simulink model "PID_DOB_sim"  (R2023b)
settings: Solver=VariableStepAuto  StartTime=0.0  StopTime=2  RelTol=1e-3
values from neighbouring files (symbols this model uses):
  Beq = Jeq/t    (= 0.00264630474582)    [PID_DOB.m]
  Beq_L = Beq+((Kg^2)*B_l/a)    (= 0.00468909971272)    [PID_DOB.m]
  Jeq = J + Kg^2/a*Jg    (= 9.9501058443e-06)    [PID_DOB.m]
  Jeq_L = Jeq+((Kg^2)*J_l/a)    (= 1.76310149198e-05)    [PID_DOB.m]
  Ka_c = 1/Kp_c    (= 1.20941973492)    [PID_DOB.m]
  Ka_s = 1/Kp_s    (= 0.380593455832)    [PID_DOB.m]
  Kd_p = wcp/wcs    (= 0.1)    [PID_DOB.m]
  Ke = Kt    (= 0.0683)    [PID_DOB.m]
  Kg = 1/81    (= 0.0123456790123)    [PID_DOB.m]
  Ki_c = Ra*wcc    (= 2211.616)    [PID_DOB.m]
  Ki_s = Beq_L*wcs/Kt*81    (= 698.796689047)    [PID_DOB.m]
  Kp_c = La*wcc    (= 0.8268428)    [PID_DOB.m]
  Kp_p = wcp    (= 12.566)    [PID_DOB.m]
  Kp_s = Jeq_L*wcs/Kt*81    (= 2.62747555082)    [PID_DOB.m]
  Kt = 68.3*10^-3    (= 0.0683)    [PID_DOB.m]
  La = 0.658*10^-3    (= 0.000658)    [PID_DOB.m]
  Ra = 1.76    [PID_DOB.m]
  tau = 0.001    [PID_DOB.m]
undefined symbols (not defined in the file or in its folder): X, Y, Z
libraries: sm_lib x8, nesl_utility x4
settings Model: Creator=OWNER  LastModifiedBy=Magnetic_Robotics
settings DebuggingCC: UnconnectedInputMsg=warning  UnconnectedOutputMsg=warning  UnconnectedLineMsg=warning
settings ModelReferenceCC: EnableRefExpFcnMdlSchedulingChecks=on
settings RTWCC: DLArmComputeVersion=19.05

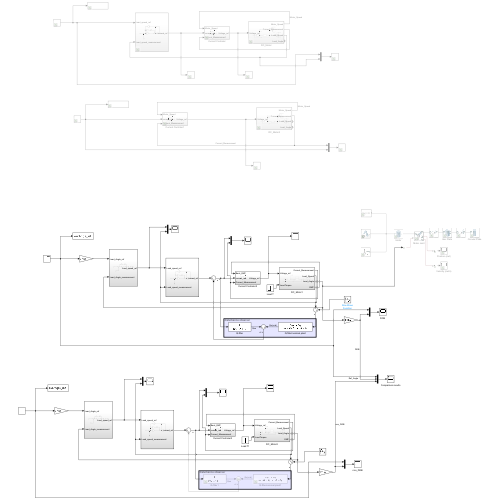
[thumbnail: Simulink's stored preview of the top-level diagram]
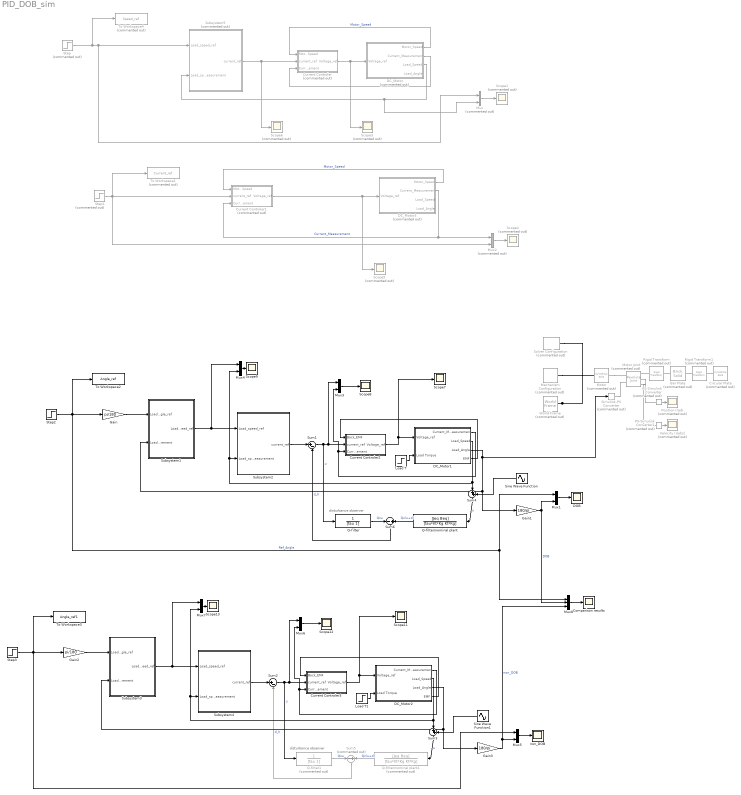
== system PID_DOB_sim ==
  note: disturbance observer
  note: disturbance observer
  Bar Plate : sm_lib/Body Elements/Brick Solid  Commented=on  GraphicAmbientColor=[0.15 0.15 0.15 1.0]  BasedOnType=Mass  BrickDimensions=[10 25 300]  BrickDimensionsUnits=mm  CenterOfMass=[0 0 0]  CenterOfMassUnits=m  GraphicDiffuseColor=[1.0 0.2 0.2]  Density=1000  DensityUnits=kg/m^3  DoExposeReferenceFrame=off  GraphicEmissiveColor=[0.0 0.0 0.0 1.0]  ExportEntireGeometry=off  SerializedFrames=<Frames><Frame><Id>Frame1</Id><Value><Name>F1</Name><Origin><Source>GeometricFeature</Source><FeatureName>-z surface</FeatureName></Origin><PrimaryAxis><DefinedDirection>+X</DefinedDirection><Source>ReferenceFrame</Source><SourceDirection>+Z</SourceDirection><FeatureName></FeatureName></PrimaryAxis><SecondaryAxis><DefinedDirection>+Z</DefinedDirection><Source>ReferenceFrame</Source><SourceDirection>+X</SourceDirection><FeatureName></FeatureName></SecondaryAxis></Value></Frame><Frame><Id>Frame2</Id><Value><Name>F2</Name><Origin><Source>GeometricFeature</Source><FeatureName>+z surface</FeatureName></Origin><PrimaryAxis><DefinedDirection>+Y</DefinedDirection><Source>ReferenceFrame</Source><SourceDirection>+Z</SourceDirection><FeatureName></FeatureName></PrimaryAxis><SecondaryAxis><DefinedDirection>+Z</DefinedDirection><Source>ReferenceFrame</Source><SourceDirection>+X</SourceDirection><FeatureName></FeatureName></SecondaryAxis></Value></Frame></Frames>  MarkerShape=Sphere  MarkerSize=10  GraphicType=FromGeometry  InertiaType=CalculateFromGeometry  Mass=175  MassUnits=g  MomentsOfInertia=[1 1 1]  MomentsOfInertiaUnits=kg*m^2  GraphicOpacity=1.0  ProductsOfInertia=[0 0 0]  ProductsOfInertiaUnits=kg*m^2  GraphicShininess=75  GraphicSpecularColor=[0.5 0.5 0.5 1.0]  GraphicVisPropType=SimpleVisualProperties
  Circular Plate : sm_lib/Body Elements/Cylindrical Solid  Commented=on  GraphicAmbientColor=[0.15 0.15 0.15 1.0]  BasedOnType=Mass  CenterOfMass=[0 0 0]  CenterOfMassUnits=m  GraphicDiffuseColor=[1.0 0.0 0.8]  CylinderLength=10  CylinderLengthUnits=mm  CylinderRadius=50  CylinderRadiusUnits=mm  Density=1000  DensityUnits=kg/m^3  DoExposeReferenceFrame=off  GraphicEmissiveColor=[0.0 0.0 0.0 1.0]  ExportEntireGeometry=off  SerializedFrames=<Frames><Frame><Id>Frame1</Id><Value><Name>F1</Name><Origin><Source>ReferenceFrame</Source><FeatureName></FeatureName></Origin><PrimaryAxis><DefinedDirection>+Z</DefinedDirection><Source>ReferenceFrame</Source><SourceDirection>+Z</SourceDirection><FeatureName></FeatureName></PrimaryAxis><SecondaryAxis><DefinedDirection>+X</DefinedDirection><Source>ReferenceFrame</Source><SourceDirection>+X</SourceDirection><FeatureName></FeatureName></SecondaryAxis></Value></Frame></Frames>  MarkerShape=Sphere  MarkerSize=10  GraphicType=FromGeometry  InertiaType=CalculateFromGeometry  Mass=340  MassUnits=g  MomentsOfInertia=[1 1 1]  MomentsOfInertiaUnits=kg*m^2  GraphicOpacity=1.0  ProductsOfInertia=[0 0 0]  ProductsOfInertiaUnits=kg*m^2  GraphicShininess=75  GraphicSpecularColor=[0.5 0.5 0.5 1.0]  GraphicVisPropType=SimpleVisualProperties
  Comparison results : Scope
  Current Controler : Subsystem  Commented=on
  Current Controler1 : Subsystem  Commented=on
  Current Controler2 : Subsystem
  Current Controler3 : Subsystem
  DC_Motor : Subsystem  Commented=on
  DC_Motor1 : Subsystem
  DC_Motor2 : Subsystem
  DC_Motor3 : Subsystem  Commented=on
  DOB : Scope
  Gain : Gain  Gain=pi/180
  Gain1 : Gain  Gain=180/pi
  Gain2 : Gain  Gain=pi/180
  Gain3 : Gain  Gain=180/pi
  Load T : Step  Time=0.1  After=2  SampleTime=0
  Load T1 : Step  Time=0.1  After=2  SampleTime=0
  Mechanism Configuration : sm_lib/Utilities/Mechanism Configuration  Commented=on  UniformGravity=Constant  GravityVector=[0 0 -9.80665]  GravityVectorUnits=m/s^2  LinearizationDelta=0.001  JointModeTransitionNonlinearIterations=2
  Motor : sm_lib/Body Elements/Cylindrical Solid  Commented=on  GraphicAmbientColor=[0.15 0.15 0.15 1.0]  BasedOnType=Density  CenterOfMass=[0 0 0]  CenterOfMassUnits=m  GraphicDiffuseColor=[0.5 0.5 0.5]  CylinderLength=150  CylinderLengthUnits=mm  CylinderRadius=30  CylinderRadiusUnits=mm  Density=1000  DensityUnits=kg/m^3  DoExposeReferenceFrame=off  GraphicEmissiveColor=[0.0 0.0 0.0 1.0]  ExportEntireGeometry=off  SerializedFrames=<Frames><Frame><Id>Frame1</Id><Value><Name>F1</Name><Origin><Source>ReferenceFrame</Source><FeatureName></FeatureName></Origin><PrimaryAxis><DefinedDirection>+Z</DefinedDirection><Source>ReferenceFrame</Source><SourceDirection>+Z</SourceDirection><FeatureName></FeatureName></PrimaryAxis><SecondaryAxis><DefinedDirection>+X</DefinedDirection><Source>ReferenceFrame</Source><SourceDirection>+X</SourceDirection><FeatureName></FeatureName></SecondaryAxis></Value></Frame><Frame><Id>Frame2</Id><Value><Name>F2</Name><Origin><Source>GeometricFeature</Source><FeatureName>top surface</FeatureName></Origin><PrimaryAxis><DefinedDirection>+Z</DefinedDirection><Source>ReferenceFrame</Source><SourceDirection>+Z</SourceDirection><FeatureName></FeatureName></PrimaryAxis><SecondaryAxis><DefinedDirection>+X</DefinedDirection><Source>ReferenceFrame</Source><SourceDirection>+X</SourceDirection><FeatureName></FeatureName></SecondaryAxis></Value></Frame></Frames>  MarkerShape=Sphere  MarkerSize=10  GraphicType=FromGeometry  InertiaType=CalculateFromGeometry  Mass=1  MassUnits=kg  MomentsOfInertia=[1 1 1]  MomentsOfInertiaUnits=kg*m^2  GraphicOpacity=1.0  ProductsOfInertia=[0 0 0]  ProductsOfInertiaUnits=kg*m^2  GraphicShininess=75  GraphicSpecularColor=[0.5 0.5 0.5 1.0]  GraphicVisPropType=SimpleVisualProperties
  Motor Joint : sm_lib/Joints/Revolute Joint  Commented=on  JointMode=Normal  SenseConstraintForce=off  SenseConstraintForceX=off  SenseConstraintForceY=off  SenseConstraintForceZ=off  SenseConstraintTorque=off  SenseConstraintTorqueX=off  SenseConstraintTorqueY=off  SenseConstraintTorqueZ=off  SenseTotalForce=off  SenseTotalForceX=off  SenseTotalForceY=off  SenseTotalForceZ=off  SenseTotalTorque=off  SenseTotalTorqueX=off  SenseTotalTorqueY=off  SenseTotalTorqueZ=off  CompositeWrenchDir=FollowerOnBase  CompositeWrenchFrame=BaseFrame  EquilibriumPosition=0  EquilibriumPositionUnits=deg  SpringStiffness=0  SpringStiffnessUnits=N*m/deg  DampingCoefficient=0  DampingCoefficientUnits=N*m/(deg/s)  TorqueActuationMode=ComputedTorque  MotionActuationMode=InputMotion  SensePosition=on  SenseVelocity=on  SenseAcceleration=off  SenseTorqueForce=off  SenseLowerLimitTorqueForce=off  SenseUpperLimitTorqueForce=off  LowerLimitSpecify=off  LowerLimitBound=-90  LowerLimitBoundUnits=deg  LowerLimitStiffness=1e4  LowerLimitStiffnessUnits=N*m/deg  LowerLimitDamping=10  LowerLimitDampingUnits=N*m/(deg/s)  LowerLimitTransitionRegionWidth=0.1  LowerLimitTransitionRegionWidthUnits=deg  UpperLimitSpecify=off  UpperLimitBound=90  UpperLimitBoundUnits=deg  UpperLimitStiffness=1e4  UpperLimitStiffnessUnits=N*m/deg  UpperLimitDamping=10  UpperLimitDampingUnits=N*m/(deg/s)  UpperLimitTransitionRegionWidth=0.1  UpperLimitTransitionRegionWidthUnits=deg  PositionTargetSpecify=off  PositionTargetPriority=High  PositionTargetValue=0  PositionTargetValueUnits=deg  VelocityTargetSpecify=off  VelocityTargetPriority=High  VelocityTargetValue=0  VelocityTargetValueUnits=deg/s
  Mux : Mux  Commented=on  Inputs=2
  Mux{1,3..7} (6 alike) : Mux  Inputs=2
  Mux2 : Mux  Commented=on  Inputs=2
  Mux8 : Mux  Inputs=3
  PS-Simulink Converter : nesl_utility/PS-Simulink Converter  Commented=on  PhysicalDomain=network_engine_domain  SubClassName=ps_output  LeftPortType=input  RightPortType=output  PseudoPeriodic=off  Frequencies=[]  VectorFormat=1-D array  Unit=inherit  AffineConversion=off
  PS-Simulink Converter1 : nesl_utility/PS-Simulink Converter  Commented=on  PhysicalDomain=network_engine_domain  SubClassName=ps_output  LeftPortType=input  RightPortType=output  PseudoPeriodic=off  Frequencies=[]  VectorFormat=1-D array  Unit=inherit  AffineConversion=off
  Position (rad) : Scope  Commented=on
  Q-filter : TransferFcn  Denominator=[tau 1]
  Q-filter/nominal plant : TransferFcn  Numerator=[Jeq Beq]  Denominator=[tau*Kt*Kg Kt*Kg]
  Q-filter/nominal plant1 : TransferFcn  Commented=on  Numerator=[Jeq Beq]  Denominator=[tau*Kt*Kg Kt*Kg]
  Q-filter1 : TransferFcn  Commented=on  Denominator=[tau 1]
  Rigid Transform : sm_lib/Frames and Transforms/Rigid Transform  Commented=on  TranslationMethod=StandardAxis  TranslationStandardOffset=5  TranslationStandardOffsetUnits=mm  TranslationStandardAxis=+Z  TranslationCartesianOffset=[0 0 0]  TranslationCartesianOffsetUnits=mm  TranslationROffset=0  TranslationROffsetUnits=m  TranslationZOffset=0  TranslationZOffsetUnits=m  TranslationThetaOffset=0  TranslationThetaOffsetUnits=deg  RotationMethod=None  RotationAngleUnits=deg  RotationStandardAxis=+Z  RotationAngle=0.0  RotationArbitraryAxis=[0 0 1]  FollAlignAxisA=+X  BaseAlignAxisA=+Y  FollAlignAxisB=+Y  BaseAlignAxisB=+Z  RotationSequenceAxes=FollowerAxes  RotationSequence=XYX  RotationSequenceAngles=[0 0 0]  RotationSequenceAnglesUnits=deg  RotationMatrix=[1 0 0; 0 1 0; 0 0 1]  Quaternion=[1 0 0 0]
  Rigid Transform1 : sm_lib/Frames and Transforms/Rigid Transform  Commented=on  TranslationMethod=StandardAxis  TranslationStandardOffset=10  TranslationStandardOffsetUnits=mm  TranslationStandardAxis=+Z  TranslationCartesianOffset=[0 0 0]  TranslationCartesianOffsetUnits=mm  TranslationROffset=0  TranslationROffsetUnits=m  TranslationZOffset=0  TranslationZOffsetUnits=m  TranslationThetaOffset=0  TranslationThetaOffsetUnits=deg  RotationMethod=None  RotationAngleUnits=deg  RotationStandardAxis=+Z  RotationAngle=0.0  RotationArbitraryAxis=[0 0 1]  FollAlignAxisA=+X  BaseAlignAxisA=+Y  FollAlignAxisB=+Y  BaseAlignAxisB=+Z  RotationSequenceAxes=FollowerAxes  RotationSequence=XYX  RotationSequenceAngles=[0 0 0]  RotationSequenceAnglesUnits=deg  RotationMatrix=[1 0 0; 0 1 0; 0 0 1]  Quaternion=[1 0 0 0]
  Scope{1,3..6} (5 alike) : Scope  Commented=on
  Scope{7..9,11..13} (6 alike) : Scope
  Simulink-PS Converter : nesl_utility/Simulink-PS Converter  Commented=on  PhysicalDomain=network_engine_domain  SubClassName=ps_input  LeftPortType=input  RightPortType=output  PseudoPeriodic=off  Frequencies=[]  NoiseDistribution=none  NoiseParameters=[]  Unit=rad  AffineConversion=off  FilteringAndDerivatives=filter  SimscapeFilterOrder=2  InputFilterTimeConstant=0.001  UdotUserProvided=0
  Sine Wave Function : Sin  Frequency=10  SampleTime=0
  Sine Wave Function1 : Sin  Frequency=10  SampleTime=0
  Solver Configuration : nesl_utility/Solver Configuration  Commented=on  PhysicalDomain=network_engine_domain  SubClassName=solver  LeftPortType=input  RightPortType=generic  Tones=[]  Harmonics=[]  SimulateNoise=off  Profile=off  UseLocalSampling=off  EnableSwitchedLinearOptims=on  FrequencyDomain=off  UseCCode=off  RelTol=0.001  AbsTol=0.001  MinStep=1e-09  ToWorkspace=off  RevertToSquareIcSolve=off  NumHomotopyIterations=100  PhasorMode=off  PhasorModeNumHarmonics=1  ConsistencySolver=NEWTON_FTOL  IndexReductionMethod=DerivativeReplacement  DoDC=off  ResidualTolerance=1e-09  ConsistencyTolSource=GLOBAL  ConsistencyAbsTol=0.001  ConsistencyRelTol=0.001  ConsistencyTolFactor=0.001  UseLocalSolver=off  LocalSolverChoice=NE_BACKWARD_EULER_ADVANCER  ResolveIndetEquations=on  FunctionEvalNumThread=1  LocalSolverSampleTime=0.001  DoFixedCost=off  MaxNonlinIter=3  MaxModeIter=2  ComputeImpulses=off  ImpulseIterations=2  LinearAlgebra=auto  LinearAlgebraNumThread=0  EquationFormulation=NE_TIME_EF  DelaysMemoryBudget=1024  AutomaticFiltering=on  FilteringTimeConstant=0.001  PartitionStorageMethod=AS_NEEDED  PartitionMemoryBudget=1024  PartitionMethod=ROBUST  MultibodyUseLocalSolver=off  MultibodyLocalSolverChoice=ODE1  MultibodyLocalSolverSampleTime=0.001
  Step : Step  Commented=on  Before=5  After=5  SampleTime=0
  Step1 : Step  Commented=on  Before=25  After=25  SampleTime=0
  Step2 : Step  Time=0.1  After=60  SampleTime=0
  Step3 : Step  Time=0.1  After=60  SampleTime=0
  Subsystem1 : Subsystem
  Subsystem2 : Subsystem
  Subsystem3 : Subsystem
  Subsystem4 : Subsystem
  Subsystem5 : Subsystem  Commented=on
  Sum1 : Sum  Inputs=|+-
  Sum2 : Sum  Inputs=|+-
  Sum3 : Sum  Inputs=|++
  Sum4 : Sum  Inputs=|++
  Sum5 : Sum  Commented=on  Inputs=-|+
  Sum6 : Sum  Inputs=-|+
  To Workspace1 : ToWorkspace  Commented=on  VariableName=Current_ref  SaveFormat=Structure With Time  SampleTime=-1
  To Workspace2 : ToWorkspace  VariableName=Angle_ref  SaveFormat=Structure With Time  SampleTime=-1
  To Workspace3 : ToWorkspace  VariableName=Angle_ref1  SaveFormat=Structure With Time  SampleTime=-1
  To Workspace4 : ToWorkspace  Commented=on  VariableName=Speed_ref  SaveFormat=Structure With Time  SampleTime=-1
  Velocity (rad/s) : Scope  Commented=on
  World Frame : sm_lib/Frames and Transforms/World Frame  Commented=on
  non_DOB : Scope
  wires:
  DC_Motor/1(Motor_Speed) -> Current Controler/1(Motor_Speed)  "Motor_Speed"
  Step/1 -> To Workspace4/1, Mux/1, Subsystem5/1(Load_speed_ref)
  Current Controler/1(Voltage_ref) -> Scope3/1, DC_Motor/1(Voltage_ref)
  Mux/1 -> Scope1/1
  Step1/1 -> To Workspace1/1, Mux2/2, Current Controler1/2(current_ref)
  Mux2/1 -> Scope4/1
  Current Controler1/1(Voltage_ref) -> Scope5/1, DC_Motor3/1(Voltage_ref)
  DC_Motor3/2(Current_Measurement) -> Mux2/1, Current Controler1/3(Current_Measurement)  "Current_Measurement"
  DC_Motor3/1(Motor_Speed) -> Current Controler1/1(Motor_Speed)  "Motor_Speed"
  DC_Motor/2(Current_Measurement) -> Current Controler/3(Current_Measurement)
  DC_Motor/3(Load_Speed) -> Mux/2, Subsystem5/2(Load_speed_measurement)
  Subsystem5/1(current_ref) -> Scope6/1, Current Controler/2(current_ref)
  Subsystem2/1(current_ref) -> Sum1/1
  DC_Motor1/2(Load_Speed) -> Sum4/1, Mux4/2, Subsystem2/2(Load_speed_measurement)
  Step2/1 -> Gain/1, Mux8/1, Mux1/1, To Workspace2/1  "Ref_Angle"
  Mux1/1 -> DOB/1
  Gain/1 -> Subsystem1/1(Load_Angle_ref)
  Gain1/1 -> Mux8/2, Mux1/2  "DOB"
  Subsystem1/1(Load_speed_ref) -> Subsystem2/1(Load_speed_ref), Mux4/1
  PS-Simulink Converter1/1 -> Velocity (rad/s)/1
  PS-Simulink Converter/1 -> Position (rad)/1
  Sum6/1 -> Sum1/2  "d_h"
  Q-filter/1 -> Sum6/1  "Qxu"
  Q-filter/nominal plant/1 -> Sum6/2  "Qx(u+d)"
  Sum1/1 -> Q-filter/1, Mux3/1, Current Controler2/2(current_ref)  "u"
  DC_Motor1/3(Load_Angle) -> Gain1/1, Subsystem1/2(Load_Angle_measurement), Simulink-PS Converter/1
  Load T/1 -> DC_Motor1/2(Load Torque)
  DC_Motor1/4(EMF) -> Current Controler2/1(Back_EMF)
  Current Controler2/1(Voltage_ref) -> Scope7/1, DC_Motor1/1(Voltage_ref)
  DC_Motor1/1(Current_Measurement) -> Mux3/2, Current Controler2/3(Current_Measurement)
  Mux3/1 -> Scope8/1
  Mux4/1 -> Scope9/1
  Sum4/1 -> Q-filter/nominal plant/1  "u"
  Sine Wave Function/1 -> Sum4/2
  Sine Wave Function1/1 -> Sum3/2
  Sum5/1 -> Sum2/2  "d_h"
  Q-filter/nominal plant1/1 -> Sum5/2  "Qx(u+d)"
  Sum3/1 -> Q-filter/nominal plant1/1  "u"
  Current Controler3/1(Voltage_ref) -> Scope11/1, DC_Motor2/1(Voltage_ref)
  Mux6/1 -> Scope12/1
  DC_Motor2/1(Current_Measurement) -> Mux6/2, Current Controler3/3(Current_Measurement)
  Load T1/1 -> DC_Motor2/2(Load Torque)
  Subsystem4/1(current_ref) -> Sum2/1
  DC_Motor2/2(Load_Speed) -> Sum3/1, Mux7/2, Subsystem4/2(Load_speed_measurement)
  DC_Motor2/3(Load_Angle) -> Gain3/1, Subsystem3/2(Load_Angle_measurement)
  Sum2/1 -> Q-filter1/1, Mux6/1, Current Controler3/2(current_ref)  "u"
  Q-filter1/1 -> Sum5/1  "Qxu"
  DC_Motor2/4(EMF) -> Current Controler3/1(Back_EMF)
  Step3/1 -> Gain2/1, Mux5/1, To Workspace3/1
  Subsystem3/1(Load_speed_ref) -> Subsystem4/1(Load_speed_ref), Mux7/1
  Mux5/1 -> non_DOB/1
  Mux7/1 -> Scope13/1
  Gain2/1 -> Subsystem3/1(Load_Angle_ref)
  Gain3/1 -> Mux8/3, Mux5/2  "non_DOB"
  Mux8/1 -> Comparison results/1
  connections:
  World Frame/RConn1 -- Solver Configuration/RConn1 -- Motor/LConn1 -- Mechanism Configuration/RConn1
  Circular Plate/LConn1 -- Rigid Transform1/RConn1
  Motor/RConn1 -- Motor Joint/LConn1
  Motor Joint/RConn2 -- PS-Simulink Converter/LConn1
  Bar Plate/LConn1 -- Rigid Transform/RConn1
  Rigid Transform1/LConn1 -- Bar Plate/RConn1
  Simulink-PS Converter/RConn1 -- Motor Joint/LConn2
  Rigid Transform/LConn1 -- Motor Joint/RConn1
  Motor Joint/RConn3 -- PS-Simulink Converter1/LConn1

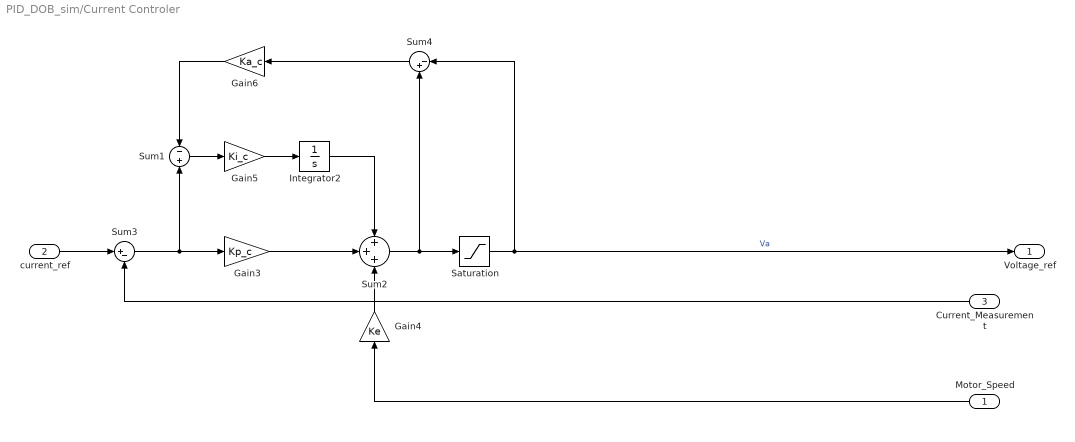
== system PID_DOB_sim/Current Controler ==
  Motor_Speed : Inport
  current_ref : Inport  Port=2
  Current_Measurement : Inport  Port=3
  Gain3 : Gain  Gain=Kp_c
  Gain4 : Gain  Gain=Ke
  Gain5 : Gain  Gain=Ki_c
  Gain6 : Gain  Gain=Ka_c
  Integrator2 : Integrator
  Saturation : Saturate  UpperLimit=48  LowerLimit=-48
  Sum1 : Sum  Inputs=-+
  Sum2 : Sum  Inputs=+++
  Sum3 : Sum  Inputs=|+-
  Sum4 : Sum  Inputs=|-+
  Voltage_ref : Outport
  wires:
  Gain6/1 -> Sum1/1
  Saturation/1 -> Voltage_ref/1, Sum4/1  "Va"
  Sum4/1 -> Gain6/1
  Sum1/1 -> Gain5/1
  Current_Measurement/1 -> Sum3/2
  Integrator2/1 -> Sum2/1
  Sum2/1 -> Sum4/2, Saturation/1
  Gain3/1 -> Sum2/2
  Gain4/1 -> Sum2/3
  Sum3/1 -> Sum1/2, Gain3/1
  Motor_Speed/1 -> Gain4/1
  Gain5/1 -> Integrator2/1
  current_ref/1 -> Sum3/1

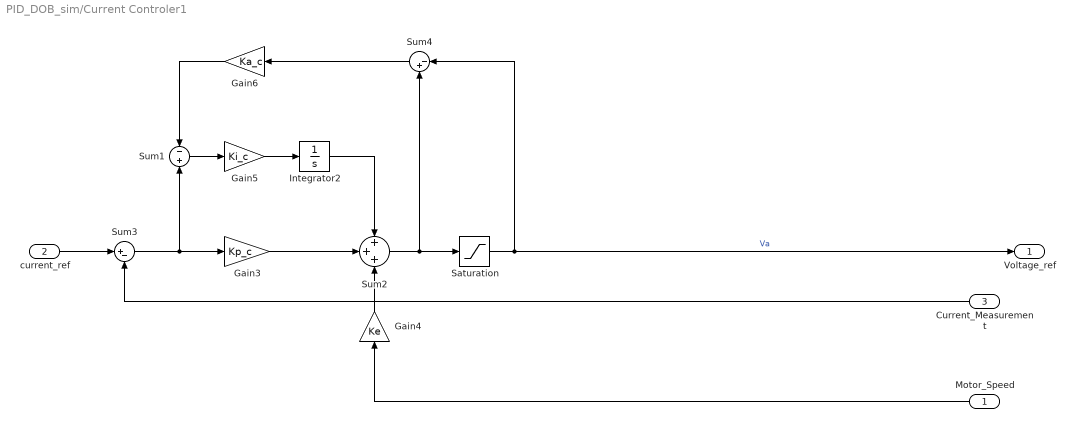
== system PID_DOB_sim/Current Controler1 ==
  Motor_Speed : Inport
  current_ref : Inport  Port=2
  Current_Measurement : Inport  Port=3
  Gain3 : Gain  Gain=Kp_c
  Gain4 : Gain  Gain=Ke
  Gain5 : Gain  Gain=Ki_c
  Gain6 : Gain  Gain=Ka_c
  Integrator2 : Integrator
  Saturation : Saturate  UpperLimit=48  LowerLimit=-48
  Sum1 : Sum  Inputs=-+
  Sum2 : Sum  Inputs=+++
  Sum3 : Sum  Inputs=|+-
  Sum4 : Sum  Inputs=|-+
  Voltage_ref : Outport
  wires:
  Gain6/1 -> Sum1/1
  Saturation/1 -> Voltage_ref/1, Sum4/1  "Va"
  Sum4/1 -> Gain6/1
  Sum1/1 -> Gain5/1
  Current_Measurement/1 -> Sum3/2
  Integrator2/1 -> Sum2/1
  Sum2/1 -> Sum4/2, Saturation/1
  Gain3/1 -> Sum2/2
  Gain4/1 -> Sum2/3
  Sum3/1 -> Sum1/2, Gain3/1
  Motor_Speed/1 -> Gain4/1
  Gain5/1 -> Integrator2/1
  current_ref/1 -> Sum3/1

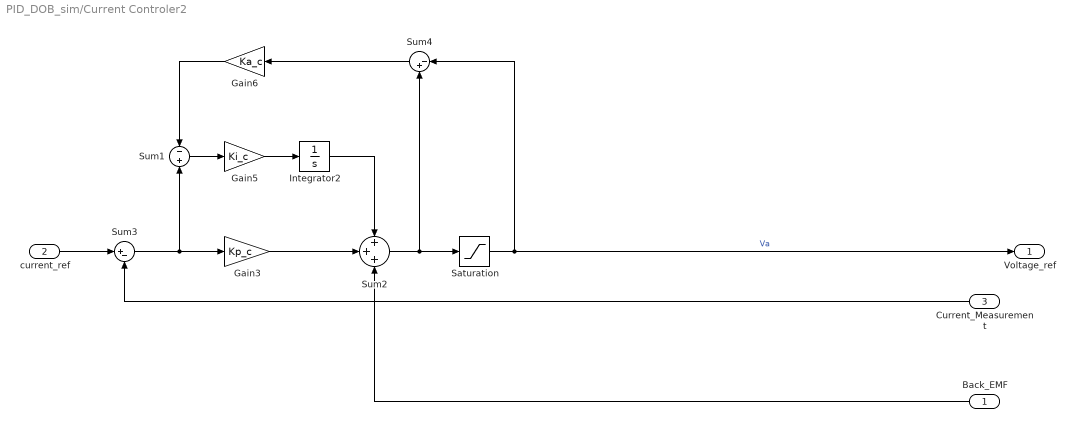
== system PID_DOB_sim/Current Controler2 ==
  Back_EMF : Inport
  current_ref : Inport  Port=2
  Current_Measurement : Inport  Port=3
  Gain3 : Gain  Gain=Kp_c
  Gain5 : Gain  Gain=Ki_c
  Gain6 : Gain  Gain=Ka_c
  Integrator2 : Integrator
  Saturation : Saturate  UpperLimit=60  LowerLimit=-60
  Sum1 : Sum  Inputs=-+
  Sum2 : Sum  Inputs=+++
  Sum3 : Sum  Inputs=|+-
  Sum4 : Sum  Inputs=|-+
  Voltage_ref : Outport
  wires:
  Gain6/1 -> Sum1/1
  Saturation/1 -> Voltage_ref/1, Sum4/1  "Va"
  Sum4/1 -> Gain6/1
  Sum1/1 -> Gain5/1
  Current_Measurement/1 -> Sum3/2
  Integrator2/1 -> Sum2/1
  Sum2/1 -> Sum4/2, Saturation/1
  Gain3/1 -> Sum2/2
  Back_EMF/1 -> Sum2/3
  Sum3/1 -> Sum1/2, Gain3/1
  Gain5/1 -> Integrator2/1
  current_ref/1 -> Sum3/1

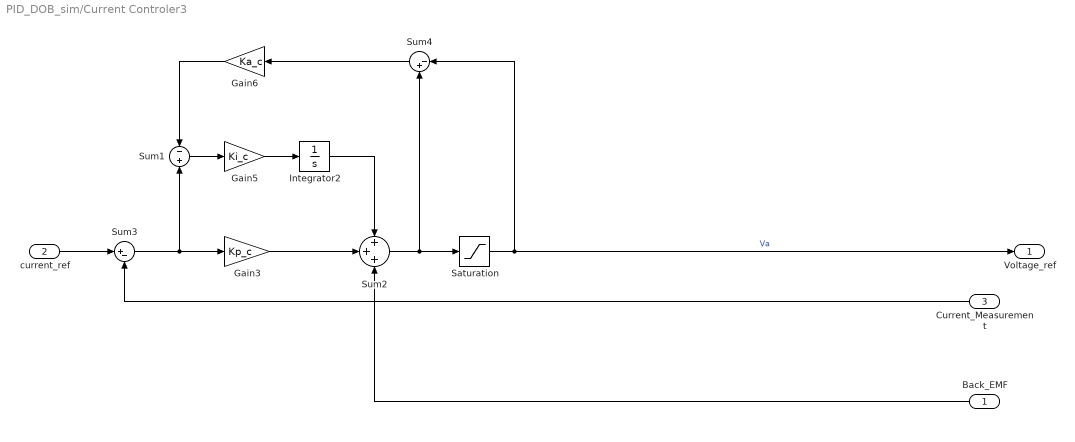
== system PID_DOB_sim/Current Controler3 ==
  Back_EMF : Inport
  current_ref : Inport  Port=2
  Current_Measurement : Inport  Port=3
  Gain3 : Gain  Gain=Kp_c
  Gain5 : Gain  Gain=Ki_c
  Gain6 : Gain  Gain=Ka_c
  Integrator2 : Integrator
  Saturation : Saturate  UpperLimit=60  LowerLimit=-60
  Sum1 : Sum  Inputs=-+
  Sum2 : Sum  Inputs=+++
  Sum3 : Sum  Inputs=|+-
  Sum4 : Sum  Inputs=|-+
  Voltage_ref : Outport
  wires:
  Gain6/1 -> Sum1/1
  Saturation/1 -> Voltage_ref/1, Sum4/1  "Va"
  Sum4/1 -> Gain6/1
  Sum1/1 -> Gain5/1
  Current_Measurement/1 -> Sum3/2
  Integrator2/1 -> Sum2/1
  Sum2/1 -> Sum4/2, Saturation/1
  Gain3/1 -> Sum2/2
  Back_EMF/1 -> Sum2/3
  Sum3/1 -> Sum1/2, Gain3/1
  Gain5/1 -> Integrator2/1
  current_ref/1 -> Sum3/1

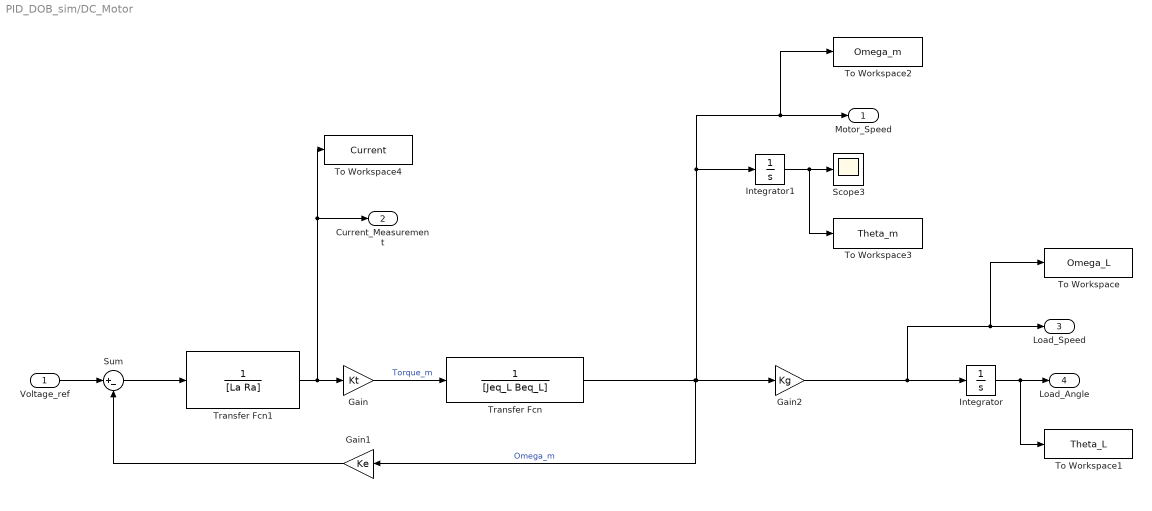
== system PID_DOB_sim/DC_Motor ==
  Voltage_ref : Inport
  Gain : Gain  Gain=Kt
  Gain1 : Gain  Gain=Ke
  Gain2 : Gain  Gain=Kg
  Integrator : Integrator
  Integrator1 : Integrator
  Scope3 : Scope
  Sum : Sum  Inputs=|+-
  To Workspace : ToWorkspace  VariableName=Omega_L  SaveFormat=Structure With Time  SampleTime=-1
  To Workspace1 : ToWorkspace  VariableName=Theta_L  SaveFormat=Structure With Time  SampleTime=-1
  To Workspace2 : ToWorkspace  VariableName=Omega_m  SaveFormat=Structure With Time  SampleTime=-1
  To Workspace3 : ToWorkspace  VariableName=Theta_m  SaveFormat=Structure With Time  SampleTime=-1
  To Workspace4 : ToWorkspace  VariableName=Current  SaveFormat=Structure With Time  SampleTime=-1
  Transfer Fcn : TransferFcn  Denominator=[Jeq_L Beq_L]
  Transfer Fcn1 : TransferFcn  Denominator=[La Ra]
  Motor_Speed : Outport
  Current_Measurement : Outport  Port=2
  Load_Speed : Outport  Port=3
  Load_Angle : Outport  Port=4
  wires:
  Voltage_ref/1 -> Sum/1
  Gain2/1 -> Load_Speed/1, To Workspace/1, Integrator/1
  Transfer Fcn/1 -> Gain2/1, Motor_Speed/1, To Workspace2/1, Integrator1/1, Gain1/1  "Omega_m"
  Gain/1 -> Transfer Fcn/1  "Torque_m"
  Transfer Fcn1/1 -> Current_Measurement/1, To Workspace4/1, Gain/1
  Integrator/1 -> Load_Angle/1, To Workspace1/1
  Gain1/1 -> Sum/2
  Integrator1/1 -> To Workspace3/1, Scope3/1
  Sum/1 -> Transfer Fcn1/1

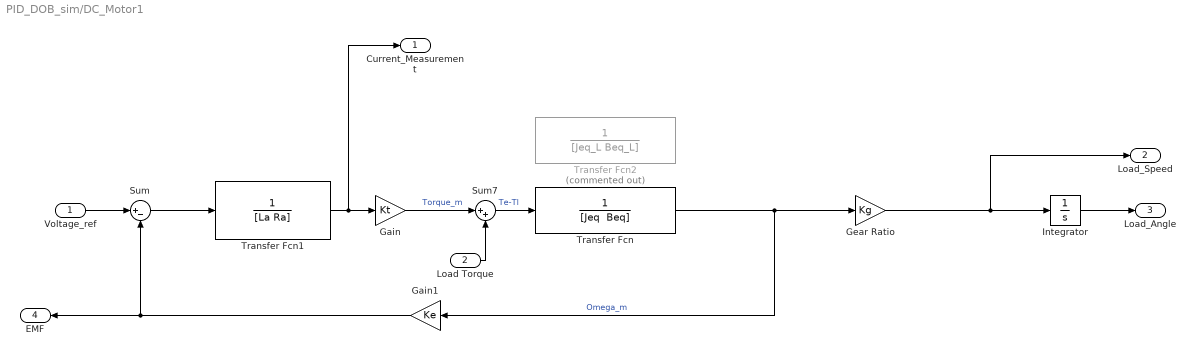
== system PID_DOB_sim/DC_Motor1 ==
  Voltage_ref : Inport
  Load Torque : Inport  Port=2
  Gain : Gain  Gain=Kt
  Gain1 : Gain  Gain=Ke
  Gear Ratio : Gain  Gain=Kg
  Integrator : Integrator
  Sum : Sum  Inputs=|+-
  Sum7 : Sum  Inputs=|++
  Transfer Fcn : TransferFcn  Denominator="[Jeq  Beq]"
  Transfer Fcn1 : TransferFcn  Denominator=[La Ra]
  Transfer Fcn2 : TransferFcn  Commented=on  Denominator=[Jeq_L Beq_L]
  Current_Measurement : Outport
  Load_Speed : Outport  Port=2
  Load_Angle : Outport  Port=3
  EMF : Outport  Port=4
  wires:
  Voltage_ref/1 -> Sum/1
  Gear Ratio/1 -> Load_Speed/1, Integrator/1
  Transfer Fcn/1 -> Gear Ratio/1, Gain1/1  "Omega_m"
  Gain/1 -> Sum7/1  "Torque_m"
  Transfer Fcn1/1 -> Current_Measurement/1, Gain/1
  Integrator/1 -> Load_Angle/1
  Gain1/1 -> Sum/2, EMF/1
  Sum/1 -> Transfer Fcn1/1
  Load Torque/1 -> Sum7/2
  Sum7/1 -> Transfer Fcn/1  "Te-Tl"

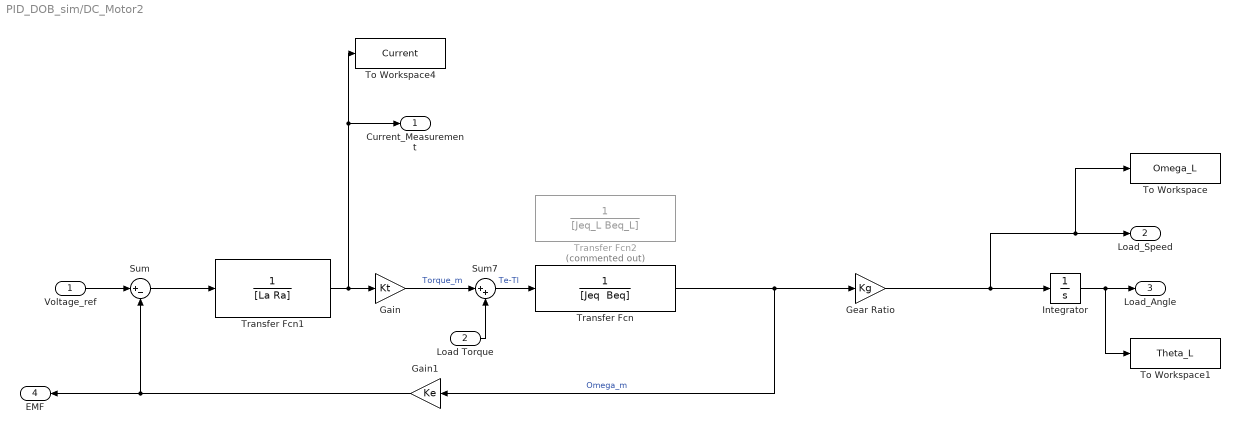
== system PID_DOB_sim/DC_Motor2 ==
  Voltage_ref : Inport
  Load Torque : Inport  Port=2
  Gain : Gain  Gain=Kt
  Gain1 : Gain  Gain=Ke
  Gear Ratio : Gain  Gain=Kg
  Integrator : Integrator
  Sum : Sum  Inputs=|+-
  Sum7 : Sum  Inputs=|++
  To Workspace : ToWorkspace  VariableName=Omega_L  SaveFormat=Structure With Time  SampleTime=-1
  To Workspace1 : ToWorkspace  VariableName=Theta_L  SaveFormat=Structure With Time  SampleTime=-1
  To Workspace4 : ToWorkspace  VariableName=Current  SaveFormat=Structure With Time  SampleTime=-1
  Transfer Fcn : TransferFcn  Denominator="[Jeq  Beq]"
  Transfer Fcn1 : TransferFcn  Denominator=[La Ra]
  Transfer Fcn2 : TransferFcn  Commented=on  Denominator=[Jeq_L Beq_L]
  Current_Measurement : Outport
  Load_Speed : Outport  Port=2
  Load_Angle : Outport  Port=3
  EMF : Outport  Port=4
  wires:
  Voltage_ref/1 -> Sum/1
  Gear Ratio/1 -> Load_Speed/1, To Workspace/1, Integrator/1
  Transfer Fcn/1 -> Gear Ratio/1, Gain1/1  "Omega_m"
  Gain/1 -> Sum7/1  "Torque_m"
  Transfer Fcn1/1 -> Current_Measurement/1, To Workspace4/1, Gain/1
  Integrator/1 -> Load_Angle/1, To Workspace1/1
  Gain1/1 -> Sum/2, EMF/1
  Sum/1 -> Transfer Fcn1/1
  Load Torque/1 -> Sum7/2
  Sum7/1 -> Transfer Fcn/1  "Te-Tl"

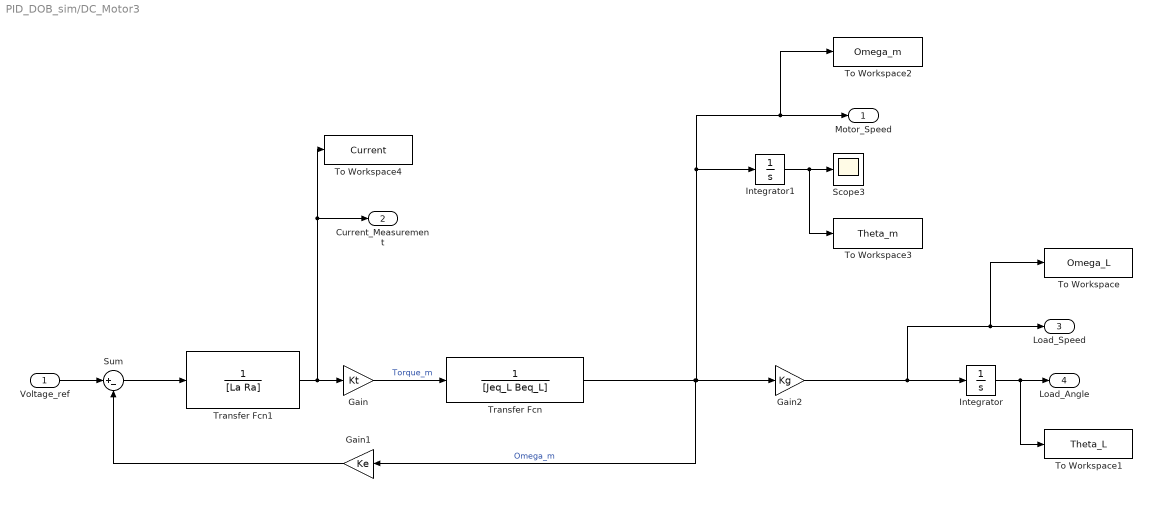
== system PID_DOB_sim/DC_Motor3 ==
  Voltage_ref : Inport
  Gain : Gain  Gain=Kt
  Gain1 : Gain  Gain=Ke
  Gain2 : Gain  Gain=Kg
  Integrator : Integrator
  Integrator1 : Integrator
  Scope3 : Scope
  Sum : Sum  Inputs=|+-
  To Workspace : ToWorkspace  VariableName=Omega_L  SaveFormat=Structure With Time  SampleTime=-1
  To Workspace1 : ToWorkspace  VariableName=Theta_L  SaveFormat=Structure With Time  SampleTime=-1
  To Workspace2 : ToWorkspace  VariableName=Omega_m  SaveFormat=Structure With Time  SampleTime=-1
  To Workspace3 : ToWorkspace  VariableName=Theta_m  SaveFormat=Structure With Time  SampleTime=-1
  To Workspace4 : ToWorkspace  VariableName=Current  SaveFormat=Structure With Time  SampleTime=-1
  Transfer Fcn : TransferFcn  Denominator=[Jeq_L Beq_L]
  Transfer Fcn1 : TransferFcn  Denominator=[La Ra]
  Motor_Speed : Outport
  Current_Measurement : Outport  Port=2
  Load_Speed : Outport  Port=3
  Load_Angle : Outport  Port=4
  wires:
  Voltage_ref/1 -> Sum/1
  Gain2/1 -> Load_Speed/1, To Workspace/1, Integrator/1
  Transfer Fcn/1 -> Gain2/1, Motor_Speed/1, To Workspace2/1, Integrator1/1, Gain1/1  "Omega_m"
  Gain/1 -> Transfer Fcn/1  "Torque_m"
  Transfer Fcn1/1 -> Current_Measurement/1, To Workspace4/1, Gain/1
  Integrator/1 -> Load_Angle/1, To Workspace1/1
  Gain1/1 -> Sum/2
  Integrator1/1 -> To Workspace3/1, Scope3/1
  Sum/1 -> Transfer Fcn1/1

== system PID_DOB_sim/Subsystem1 ==
  Load_Angle_ref : Inport
  Load_Angle_measurement : Inport  Port=2
  Derivative : Derivative
  Gain : Gain  Gain=Kd_p
  Gain1 : Gain  Gain=Kp_p
  Saturation : Saturate  UpperLimit=642.98  LowerLimit=-642.98
  Sum : Sum  Inputs=|+-
  Sum1 : Sum  Inputs=++|
  Load_speed_ref : Outport  VectorParamsAs1DForOutWhenUnconnected=off
  wires:
  Gain1/1 -> Sum1/2
  Derivative/1 -> Sum1/1
  Sum1/1 -> Saturation/1
  Sum/1 -> Gain/1, Gain1/1
  Gain/1 -> Derivative/1
  Saturation/1 -> Load_speed_ref/1
  Load_Angle_ref/1 -> Sum/1
  Load_Angle_measurement/1 -> Sum/2

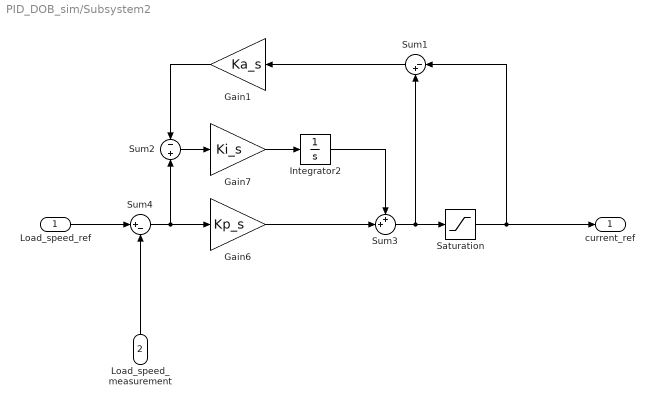
== system PID_DOB_sim/Subsystem2 ==
  Load_speed_ref : Inport
  Load_speed_measurement : Inport  Port=2
  Gain1 : Gain  Gain=Ka_s
  Gain6 : Gain  Gain=Kp_s
  Gain7 : Gain  Gain=Ki_s
  Integrator2 : Integrator
  Saturation : Saturate  UpperLimit=27.3  LowerLimit=-27.3
  Sum1 : Sum  Inputs=|-+
  Sum2 : Sum  Inputs=-|+
  Sum3 : Sum  Inputs=++|
  Sum4 : Sum  Inputs=|+-
  current_ref : Outport  VectorParamsAs1DForOutWhenUnconnected=off
  wires:
  Load_speed_measurement/1 -> Sum4/2
  Integrator2/1 -> Sum3/1
  Sum3/1 -> Sum1/2, Saturation/1
  Gain6/1 -> Sum3/2
  Gain7/1 -> Integrator2/1
  Load_speed_ref/1 -> Sum4/1
  Gain1/1 -> Sum2/1
  Sum1/1 -> Gain1/1
  Saturation/1 -> current_ref/1, Sum1/1
  Sum2/1 -> Gain7/1
  Sum4/1 -> Sum2/2, Gain6/1

== system PID_DOB_sim/Subsystem3 ==
  Load_Angle_ref : Inport
  Load_Angle_measurement : Inport  Port=2
  Derivative : Derivative
  Gain : Gain  Gain=Kd_p
  Gain1 : Gain  Gain=Kp_p
  Saturation : Saturate  UpperLimit=642.98  LowerLimit=-642.98
  Sum : Sum  Inputs=|+-
  Sum1 : Sum  Inputs=++|
  Load_speed_ref : Outport  VectorParamsAs1DForOutWhenUnconnected=off
  wires:
  Gain1/1 -> Sum1/2
  Derivative/1 -> Sum1/1
  Sum1/1 -> Saturation/1
  Sum/1 -> Gain/1, Gain1/1
  Gain/1 -> Derivative/1
  Saturation/1 -> Load_speed_ref/1
  Load_Angle_ref/1 -> Sum/1
  Load_Angle_measurement/1 -> Sum/2

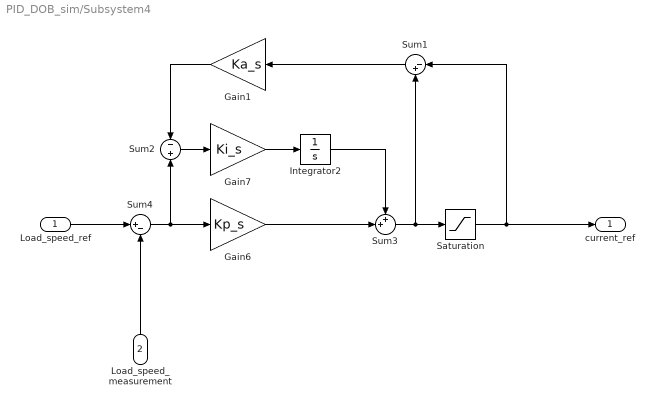
== system PID_DOB_sim/Subsystem4 ==
  Load_speed_ref : Inport
  Load_speed_measurement : Inport  Port=2
  Gain1 : Gain  Gain=Ka_s
  Gain6 : Gain  Gain=Kp_s
  Gain7 : Gain  Gain=Ki_s
  Integrator2 : Integrator
  Saturation : Saturate  UpperLimit=27.3  LowerLimit=-27.3
  Sum1 : Sum  Inputs=|-+
  Sum2 : Sum  Inputs=-|+
  Sum3 : Sum  Inputs=++|
  Sum4 : Sum  Inputs=|+-
  current_ref : Outport  VectorParamsAs1DForOutWhenUnconnected=off
  wires:
  Load_speed_measurement/1 -> Sum4/2
  Integrator2/1 -> Sum3/1
  Sum3/1 -> Sum1/2, Saturation/1
  Gain6/1 -> Sum3/2
  Gain7/1 -> Integrator2/1
  Load_speed_ref/1 -> Sum4/1
  Gain1/1 -> Sum2/1
  Sum1/1 -> Gain1/1
  Saturation/1 -> current_ref/1, Sum1/1
  Sum2/1 -> Gain7/1
  Sum4/1 -> Sum2/2, Gain6/1

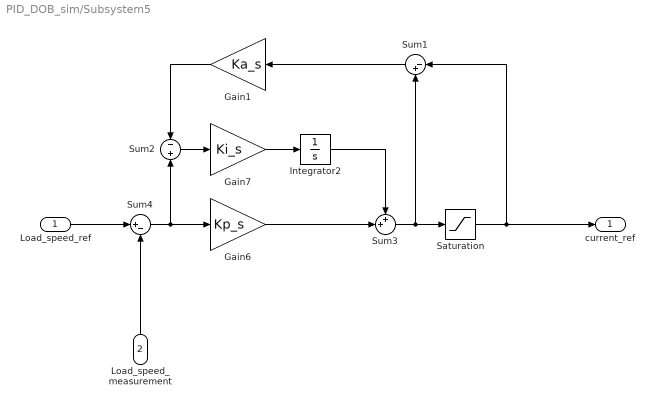
== system PID_DOB_sim/Subsystem5 ==
  Load_speed_ref : Inport
  Load_speed_measurement : Inport  Port=2
  Gain1 : Gain  Gain=Ka_s
  Gain6 : Gain  Gain=Kp_s
  Gain7 : Gain  Gain=Ki_s
  Integrator2 : Integrator
  Saturation : Saturate  UpperLimit=27.3  LowerLimit=-27.3
  Sum1 : Sum  Inputs=|-+
  Sum2 : Sum  Inputs=-|+
  Sum3 : Sum  Inputs=++|
  Sum4 : Sum  Inputs=|+-
  current_ref : Outport  VectorParamsAs1DForOutWhenUnconnected=off
  wires:
  Load_speed_measurement/1 -> Sum4/2
  Integrator2/1 -> Sum3/1
  Sum3/1 -> Sum1/2, Saturation/1
  Gain6/1 -> Sum3/2
  Gain7/1 -> Integrator2/1
  Load_speed_ref/1 -> Sum4/1
  Gain1/1 -> Sum2/1
  Sum1/1 -> Gain1/1
  Saturation/1 -> current_ref/1, Sum1/1
  Sum2/1 -> Gain7/1
  Sum4/1 -> Sum2/2, Gain6/1
